simulink model "EIS_Blei_pos_Konz"  (Simulink 9.0)
settings: Solver=ode45  StartTime=0.0  StopTime=t_end  FixedStep=1/sample/f/10  MaxStep=1/sample/f/11  MinStep=1/sample/f/1e12  RelTol=1e-12  AbsTol=1e-15  EnableMultiTasking=on
values from neighbouring files (symbols this model uses):
  Cdl = 6000    [Blei_pos_Konz.m]
  conc_f = conc_Pb(fi,n)    [Blei_pos_Konz.m]
  conc_SO = conc_SO4(fi,n)    [Blei_pos_Konz.m]
  electrode = 1    [Blei_pos_Konz.m]
  F = 96487    [Blei_pos_Konz.m]
  f = frequency(fi)    [Blei_pos_Konz.m]
  I = I_DC(n)    [Blei_pos_Konz.m]
  isin = isinus    (= 0.01)    [Blei_pos_Konz.m]
  L = 1e-8    (= 1e-08)    [Blei_pos_Konz.m]
  R = 8.3145    [Blei_pos_Konz.m]
  R1 = 0.05e-3    (= 5e-05)    [Blei_pos_Konz.m]
  R2 = 0.05e-3    (= 5e-05)    [Blei_pos_Konz.m]
  sample = 2^5    (= 32)    [Blei_pos_Konz.m]
  T = 298    [Blei_pos_Konz.m]
  U0 = 0    [Blei_pos_Konz.m]
  U_RC0 = u_RCo(end)    [Blei_pos_Konz.m]
undefined symbols (not defined in the file): pR
settings Model: Creator=sf  LastModifiedBy=JuliaKowal
settings SolverCC: InitialStep=1/sample/f/1e12  MaxOrder=1
settings DataIOCC: SignalLoggingSaveFormat=ModelDataLogs  SaveOutput=off  SignalLogging=off  SaveTime=off
settings OptimizationCC: ExpressionDepthLimit=2147483647  InitFltsAndDblsToZero=on
settings DebuggingCC: SaveWithParameterizedLinksMsg=none  SignalResolutionControl=TryResolveAllWithWarning  SolverPrmCheckMsg=warning  InheritedTsInSrcMsg=none  MultiTaskDSMMsg=warning  MultiTaskCondExecSysMsg=none  FcnCallInpInsideContextMsg=warning  StateNameClashWarn=warning  StrictBusMsg=Warning
settings GRTTargetCC: TargetFcnLib=ansi_tfl_tmw.mat  CombineOutputUpdateFcns=off  GRTInterface=on

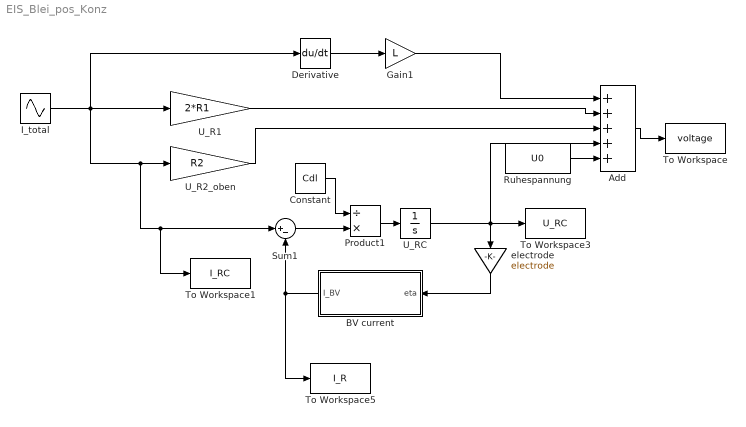
== system EIS_Blei_pos_Konz ==
  Add : Sum  Inputs=+++++
  BV current : Subsystem  mask{alpha=pR(1), I0=pR(2)}
      mask prompts: I0 "I_0"
  Constant : Constant  Value=Cdl
  Derivative : Derivative
  Gain1 : Gain  Gain=L
  I_total : Sin  Amplitude=isin  Bias=I  Frequency=2*pi*f
  Product1 : Product  Inputs=/*  RndMeth=Zero
  Ruhespannung : Constant  Value=U0
  Sum1 : Sum  Inputs=|+-
  To Workspace : ToWorkspace  VariableName=voltage  SampleTime=1/(sample*f)
  To Workspace1 : ToWorkspace  VariableName=I_RC  SampleTime=1/(sample*f)
  To Workspace3 : ToWorkspace  VariableName=U_RC  SampleTime=1/(sample*f)
  To Workspace5 : ToWorkspace  VariableName=I_R  SampleTime=1/(sample*f)
  U_R1 : Gain  Gain=2*R1
  U_R2_oben : Gain  Gain=R2
  U_RC : Integrator  InitialCondition=U_RC0
  electrode : Gain  Gain=electrode
  wires:
  I_total/1 -> U_R1/1, U_R2_oben/1, Sum1/1, To Workspace1/1, Derivative/1
  U_R1/1 -> Add/2
  Add/1 -> To Workspace/1
  U_R2_oben/1 -> Add/3
  Ruhespannung/1 -> Add/5
  U_RC/1 -> electrode/1, To Workspace3/1, Add/4
  Product1/1 -> U_RC/1
  Sum1/1 -> Product1/2
  BV current/1(I_BV) -> Sum1/2, To Workspace5/1
  Constant/1 -> Product1/1
  electrode/1 -> BV current/1(eta)
  Derivative/1 -> Gain1/1
  Gain1/1 -> Add/1

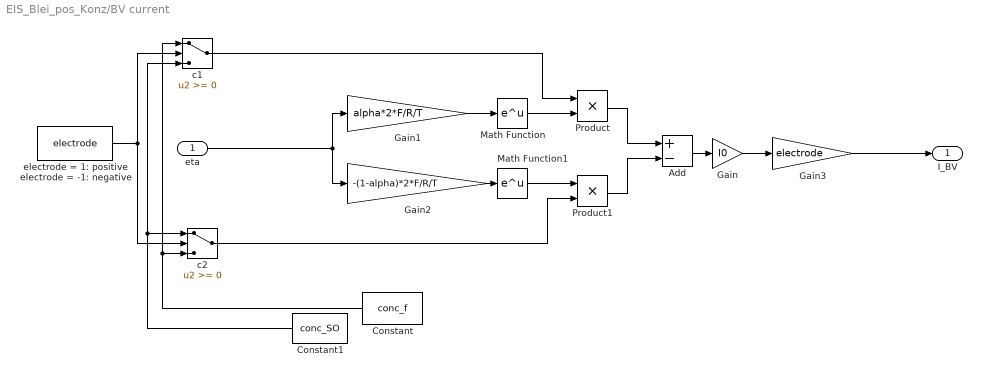
== system EIS_Blei_pos_Konz/BV current ==
  eta : Inport
  Add : Sum  Inputs=+-
  Constant : Constant  Value=conc_f
  Constant1 : Constant  Value=conc_SO
  Gain : Gain  Gain=I0
  Gain1 : Gain  Gain=alpha*2*F/R/T
  Gain2 : Gain  Gain=-(1-alpha)*2*F/R/T
  Gain3 : Gain  Gain=electrode
  Math Function : Math  SaturateOnIntegerOverflow=on
  Math Function1 : Math  SaturateOnIntegerOverflow=on
  Product : Product  RndMeth=Zero
  Product1 : Product  RndMeth=Zero
  c1 : Switch
  c2 : Switch
  electrode = 1: positive electrode = -1: negative : Constant  Value=electrode
  I_BV : Outport
  wires:
  Add/1 -> Gain/1
  Gain/1 -> Gain3/1
  Math Function/1 -> Product/2
  Product/1 -> Add/1
  Product1/1 -> Add/2
  Math Function1/1 -> Product1/1
  c1/1 -> Product/1
  c2/1 -> Product1/2
  Gain1/1 -> Math Function/1
  Gain2/1 -> Math Function1/1
  eta/1 -> Gain1/1, Gain2/1
  electrode = 1: positive electrode = -1: negative/1 -> c2/2, c1/2
  Gain3/1 -> I_BV/1
  Constant1/1 -> c2/1, c1/3
  Constant/1 -> c2/3, c1/1
